simulink model "myverify2"  (R2019a)
settings: Solver=VariableStepAuto  StartTime=0.0  StopTime=10.0  RelTol=1e-3
values from neighbouring files (symbols this model uses):
  den1 = cell2mat(Model_tf_c.den)    [main.m]
  num1 = cell2mat(Model_tf_c.num)    [main.m]
undefined symbols (not defined in the file or in its folder): a, A, b, Href
libraries: simulink x4, slident x1
settings Model: Creator=lzr96  LastModifiedBy=lzr96

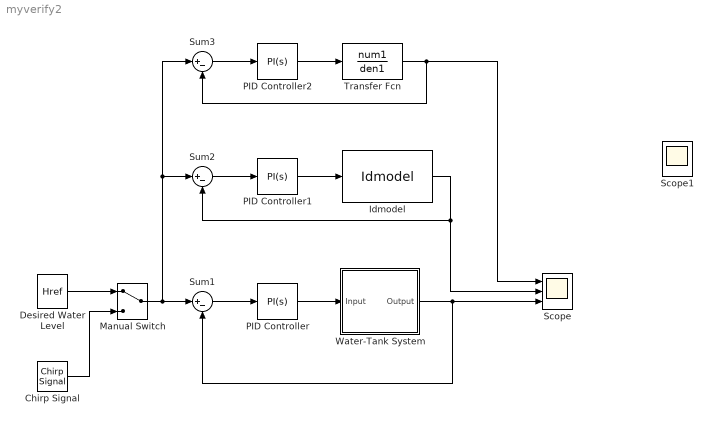
== system myverify2 ==
  Chirp Signal : simulink/Sources/Chirp Signal  f1=0.0001  T=100  f2=0.05
  Desired Water Level : Constant  Value=Href
  Idmodel : slident/Models/Idmodel  sys=Model  IC=0  noi=on  seed=[]
      settings: SourceProductName=System Identification Toolbox  SourceProductBaseCode=ID
  Manual Switch : ManualSwitch
  PID Controller : simulink/Continuous/PID Controller  Tag=PID1  Controller=PI  Form=Parallel  TimeDomain=Continuous-time  SampleTime=-1  IntegratorMethod=Forward Euler  FilterMethod=Forward Euler  ControllerParametersSource=internal  P=3.08768043183519  I=0.280839228677788  D=-7.525674  UseFilter=on  N=0.201208  TunerSelectOption=Transfer Function Based (PID Tuner App)  ZeroCross=off  InitialConditionSource=internal  InitialConditionForIntegrator=0  InitialConditionForFilter=0  DifferentiatorICPrevScaledInput=0  ExternalReset=none  TrackingMode=off  Kt=1  LimitOutput=off  UpperSaturationLimit=inf  LowerSaturationLimit=-inf  LinearizeAsGain=off  AntiWindupMode=none  Kb=1  POutMin=[ ]  POutMax=[ ]  IOutMin=[ ]  IOutMax=[ ]  DOutMin=[ ]  DOutMax=[ ]  NOutMin=[ ]  NOutMax=[ ]  SumOutMin=[ ]  SumOutMax=[ ]  SaturationOutMin=[ ]  SaturationOutMax=[ ]  PParamMin=[ ]  PParamMax=[ ]  IParamMin=[ ]  IParamMax=[ ]  DParamMin=[ ]  DParamMax=[ ]  NParamMin=[ ]  NParamMax=[ ]  KbParamMin=[ ]  KbParamMax=[ ]  KtParamMin=[ ]  KtParamMax=[ ]  KbOutMin=[ ]  KbOutMax=[ ]  KtOutMin=[ ]  KtOutMax=[ ]  IntegratorOutMin=[ ]  IntegratorOutMax=[ ]  FilterOutMin=[ ]  FilterOutMax=[ ]  SumI1OutMin=[ ]  SumI1OutMax=[ ]  SumI2OutMin=[ ]  SumI2OutMax=[ ]  SumI3OutMin=[ ]  SumI3OutMax=[ ]  SumI4OutMin=[]  SumI4OutMax=[]  SumDOutMin=[ ]  SumDOutMax=[ ]  DifferentiatorOutMin=[]  DifferentiatorOutMax=[]  FilterDiffOutCoefMin=[]  FilterDiffOutCoefMax=[]  ReciprocalOutMin=[]  ReciprocalOutMax=[]  SumDenOutMin=[]  SumDenOutMax=[]  SumNumOutMin=[]  SumNumOutMax=[]  DivideOutMin=[]  DivideOutMax=[]  IntegratorContinuousStateAttributes=''  IntegratorStateMustResolveToSignalObject=off  IntegratorRTWStateStorageClass=Auto  FilterContinuousStateAttributes=''  FilterStateMustResolveToSignalObject=off  FilterRTWStateStorageClass=Auto  ParallelPVariant=InternalParameters  IdealPVariant=Disabled  IVariant=InternalParameters  DVariant=Disabled  IntegratorVariant=Continuous  SatVariant=Disabled  AWVariant=Passthrough  PCopyVariant=Disabled  TRVariant=Disabled  FdbkBlocksVariant=Forward  IdealPFdbkVariant=Disabled  SatFdbkVariant=Disabled  DerivativeFilterVariant=Disabled  NVariant=Disabled  NCopyVariant=Disabled_SignalSpec  FilterICVariant=Disabled  IntegratorICVariant=InternalICs  ExternalResetVariant=Disabled  TRSumVariant=Passthrough  SumFdbkVariant=Disabled  SumVariant=Sum_PI
  PID Controller1 : simulink/Continuous/PID Controller  Tag=PID1  Controller=PI  Form=Parallel  TimeDomain=Continuous-time  SampleTime=-1  IntegratorMethod=Forward Euler  FilterMethod=Forward Euler  ControllerParametersSource=internal  P=3.08768043183519  I=0.280839228677788  D=-7.525674  UseFilter=on  N=0.201208  TunerSelectOption=Transfer Function Based (PID Tuner App)  ZeroCross=off  InitialConditionSource=internal  InitialConditionForIntegrator=0  InitialConditionForFilter=0  DifferentiatorICPrevScaledInput=0  ExternalReset=none  TrackingMode=off  Kt=1  LimitOutput=off  UpperSaturationLimit=inf  LowerSaturationLimit=-inf  LinearizeAsGain=off  AntiWindupMode=none  Kb=1  POutMin=[ ]  POutMax=[ ]  IOutMin=[ ]  IOutMax=[ ]  DOutMin=[ ]  DOutMax=[ ]  NOutMin=[ ]  NOutMax=[ ]  SumOutMin=[ ]  SumOutMax=[ ]  SaturationOutMin=[ ]  SaturationOutMax=[ ]  PParamMin=[ ]  PParamMax=[ ]  IParamMin=[ ]  IParamMax=[ ]  DParamMin=[ ]  DParamMax=[ ]  NParamMin=[ ]  NParamMax=[ ]  KbParamMin=[ ]  KbParamMax=[ ]  KtParamMin=[ ]  KtParamMax=[ ]  KbOutMin=[ ]  KbOutMax=[ ]  KtOutMin=[ ]  KtOutMax=[ ]  IntegratorOutMin=[ ]  IntegratorOutMax=[ ]  FilterOutMin=[ ]  FilterOutMax=[ ]  SumI1OutMin=[ ]  SumI1OutMax=[ ]  SumI2OutMin=[ ]  SumI2OutMax=[ ]  SumI3OutMin=[ ]  SumI3OutMax=[ ]  SumI4OutMin=[]  SumI4OutMax=[]  SumDOutMin=[ ]  SumDOutMax=[ ]  DifferentiatorOutMin=[]  DifferentiatorOutMax=[]  FilterDiffOutCoefMin=[]  FilterDiffOutCoefMax=[]  ReciprocalOutMin=[]  ReciprocalOutMax=[]  SumDenOutMin=[]  SumDenOutMax=[]  SumNumOutMin=[]  SumNumOutMax=[]  DivideOutMin=[]  DivideOutMax=[]  IntegratorContinuousStateAttributes=''  IntegratorStateMustResolveToSignalObject=off  IntegratorRTWStateStorageClass=Auto  FilterContinuousStateAttributes=''  FilterStateMustResolveToSignalObject=off  FilterRTWStateStorageClass=Auto  ParallelPVariant=InternalParameters  IdealPVariant=Disabled  IVariant=InternalParameters  DVariant=Disabled  IntegratorVariant=Continuous  SatVariant=Disabled  AWVariant=Passthrough  PCopyVariant=Disabled  TRVariant=Disabled  FdbkBlocksVariant=Forward  IdealPFdbkVariant=Disabled  SatFdbkVariant=Disabled  DerivativeFilterVariant=Disabled  NVariant=Disabled  NCopyVariant=Disabled_SignalSpec  FilterICVariant=Disabled  IntegratorICVariant=InternalICs  ExternalResetVariant=Disabled  TRSumVariant=Passthrough  SumFdbkVariant=Disabled  SumVariant=Sum_PI
  PID Controller2 : simulink/Continuous/PID Controller  Tag=PID1  Controller=PI  Form=Parallel  TimeDomain=Continuous-time  SampleTime=-1  IntegratorMethod=Forward Euler  FilterMethod=Forward Euler  ControllerParametersSource=internal  P=3.08768043183519  I=0.280839228677788  D=-7.525674  UseFilter=on  N=0.201208  TunerSelectOption=Transfer Function Based (PID Tuner App)  ZeroCross=off  InitialConditionSource=internal  InitialConditionForIntegrator=0  InitialConditionForFilter=0  DifferentiatorICPrevScaledInput=0  ExternalReset=none  TrackingMode=off  Kt=1  LimitOutput=off  UpperSaturationLimit=inf  LowerSaturationLimit=-inf  LinearizeAsGain=off  AntiWindupMode=none  Kb=1  POutMin=[ ]  POutMax=[ ]  IOutMin=[ ]  IOutMax=[ ]  DOutMin=[ ]  DOutMax=[ ]  NOutMin=[ ]  NOutMax=[ ]  SumOutMin=[ ]  SumOutMax=[ ]  SaturationOutMin=[ ]  SaturationOutMax=[ ]  PParamMin=[ ]  PParamMax=[ ]  IParamMin=[ ]  IParamMax=[ ]  DParamMin=[ ]  DParamMax=[ ]  NParamMin=[ ]  NParamMax=[ ]  KbParamMin=[ ]  KbParamMax=[ ]  KtParamMin=[ ]  KtParamMax=[ ]  KbOutMin=[ ]  KbOutMax=[ ]  KtOutMin=[ ]  KtOutMax=[ ]  IntegratorOutMin=[ ]  IntegratorOutMax=[ ]  FilterOutMin=[ ]  FilterOutMax=[ ]  SumI1OutMin=[ ]  SumI1OutMax=[ ]  SumI2OutMin=[ ]  SumI2OutMax=[ ]  SumI3OutMin=[ ]  SumI3OutMax=[ ]  SumI4OutMin=[]  SumI4OutMax=[]  SumDOutMin=[ ]  SumDOutMax=[ ]  DifferentiatorOutMin=[]  DifferentiatorOutMax=[]  FilterDiffOutCoefMin=[]  FilterDiffOutCoefMax=[]  ReciprocalOutMin=[]  ReciprocalOutMax=[]  SumDenOutMin=[]  SumDenOutMax=[]  SumNumOutMin=[]  SumNumOutMax=[]  DivideOutMin=[]  DivideOutMax=[]  IntegratorContinuousStateAttributes=''  IntegratorStateMustResolveToSignalObject=off  IntegratorRTWStateStorageClass=Auto  FilterContinuousStateAttributes=''  FilterStateMustResolveToSignalObject=off  FilterRTWStateStorageClass=Auto  ParallelPVariant=InternalParameters  IdealPVariant=Disabled  IVariant=InternalParameters  DVariant=Disabled  IntegratorVariant=Continuous  SatVariant=Disabled  AWVariant=Passthrough  PCopyVariant=Disabled  TRVariant=Disabled  FdbkBlocksVariant=Forward  IdealPFdbkVariant=Disabled  SatFdbkVariant=Disabled  DerivativeFilterVariant=Disabled  NVariant=Disabled  NCopyVariant=Disabled_SignalSpec  FilterICVariant=Disabled  IntegratorICVariant=InternalICs  ExternalResetVariant=Disabled  TRSumVariant=Passthrough  SumFdbkVariant=Disabled  SumVariant=Sum_PI
  Scope : Scope  NumInputPorts=3
  Scope1 : Scope  NumInputPorts=2
  Sum1 : Sum  Inputs=|+-  SaturateOnIntegerOverflow=on
  Sum2 : Sum  Inputs=|+-  SaturateOnIntegerOverflow=on
  Sum3 : Sum  Inputs=|+-  SaturateOnIntegerOverflow=on
  Transfer Fcn : TransferFcn  Numerator=num1  Denominator=den1
  Water-Tank System : Subsystem
      mask Display: image('1.bmp');
  wires:
  Desired Water Level/1 -> Manual Switch/1
  PID Controller/1 -> Water-Tank System/1(Input)
  Sum1/1 -> PID Controller/1
  Water-Tank System/1(Output) -> Sum1/2, Scope/3
  Chirp Signal/1 -> Manual Switch/2
  Manual Switch/1 -> Sum1/1, Sum2/1, Sum3/1
  Sum2/1 -> PID Controller1/1
  Idmodel/1 -> Scope/2, Sum2/2
  PID Controller1/1 -> Idmodel/1
  Sum3/1 -> PID Controller2/1
  Transfer Fcn/1 -> Sum3/2, Scope/1
  PID Controller2/1 -> Transfer Fcn/1

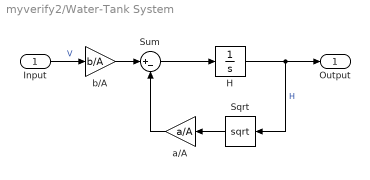
== system myverify2/Water-Tank System ==
  Input : Inport
  H : Integrator  InitialCondition=1
  Sqrt : Sqrt  OutputSignalType=real  SaturateOnIntegerOverflow=on
  Sum : Sum  Inputs=|+-  SaturateOnIntegerOverflow=on
  a/A : Gain  Gain=a/A  SaturateOnIntegerOverflow=on  OutDataTypeStr=Inherit: Same as input  ParamDataTypeStr=Inherit: Same as input
  b/A : Gain  Gain=b/A  SaturateOnIntegerOverflow=on  OutDataTypeStr=Inherit: Same as input  ParamDataTypeStr=Inherit: Same as input
  Output : Outport
  wires:
  b/A/1 -> Sum/1
  Sum/1 -> H/1
  H/1 -> Sqrt/1, Output/1  "H"
  Sqrt/1 -> a/A/1
  a/A/1 -> Sum/2
  Input/1 -> b/A/1  "V"
